simulink model "DaviAraujo_FuelHeatingModel_DashBoardOK"  (R2021a)
settings: Solver=ode5  StartTime=0.0  StopTime=inf  FixedStep=0.01  RelTol=1e-3
values from neighbouring files (symbols this model uses):
  A = 0.0003*4    (= 0.0012)    [FuelHeatingModel_WS.m]
  Densidade_Combustivel = 0.774    [FuelHeatingModel_WS.m]
  EngineTemp = 90    [FuelHeatingModel_WS.m]
  Fluxo_Injetor = 2.141967    [FuelHeatingModel_WS.m]
  h = 12000    [FuelHeatingModel_WS.m]
  Lead_MaxTemp = 80    [FuelHeatingModel_WS.m]
  LeadAcid_TotalEnergy = Voltage_LeadAcid*AmpHour_LeadAcid    (= 600)    [FuelHeatingModel_WS.m]
  Lithium_MaxTemp = 80    [FuelHeatingModel_WS.m]
  Lithium_TotalEnergy = Voltage_Lithium*AmpHour_Lithium    (= 768)    [FuelHeatingModel_WS.m]
  m = (0.4*0.79)    (= 0.316)    [FuelHeatingModel_WS.m]
  Pressure_Ethanol = (P_min:((P_max-P_min)/20):P_max).^4.92    [FuelHeatingModel_WS.m]
  PWM = 0:5:100    [FuelHeatingModel_WS.m]
  RPM_Motor = 1000    [FuelHeatingModel_WS.m]
  Setpoint_ColdStart = 120    [FuelHeatingModel_WS.m]
  Setpoint_PostStart = 90    [FuelHeatingModel_WS.m]
  Temp_Ethanol = 0:6:120    [FuelHeatingModel_WS.m]
  Ts = (Ts_min:((Ts_max-Ts_min)/20):Ts_max).^0.7    [FuelHeatingModel_WS.m]
  VolumeInterno_CommonRail = 7000    [FuelHeatingModel_WS.m]
libraries: simulink x4
(part 1 of 2)
settings Model: NumberOfSteps=10  EnablePacing=on  PacingRate=10  Creator=davi_  LastModifiedBy=davi_
settings SolverCC: AlgebraicLoopSolver=TrustRegion

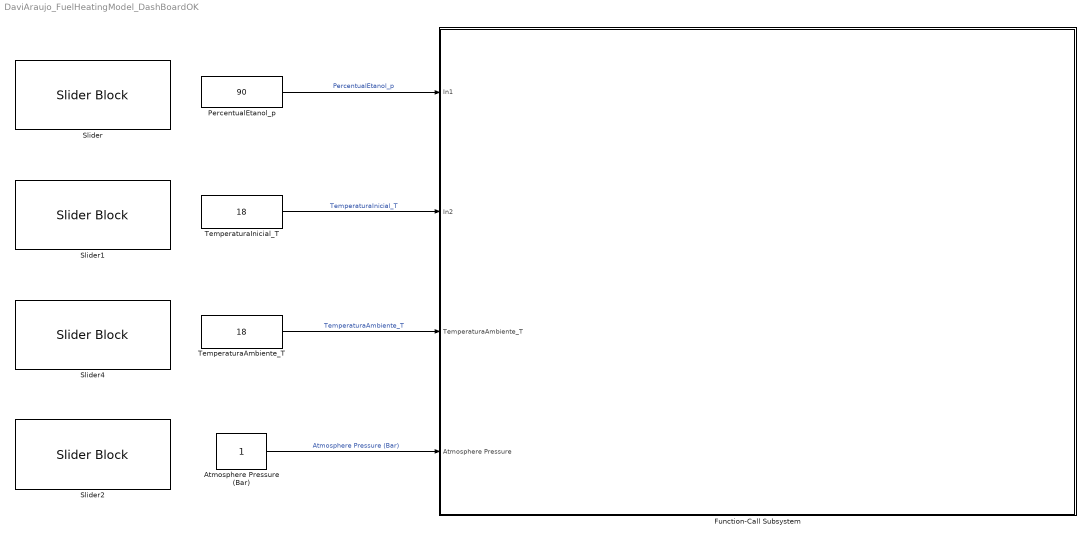
== system DaviAraujo_FuelHeatingModel_DashBoardOK ==
  Atmosphere Pressure (Bar) : Constant
  Function-Call Subsystem : Subsystem  TreatAsAtomicUnit=on
  PercentualEtanol_p : Constant  Value=90
  Slider : SliderBlock
  Slider1 : SliderBlock  ScaleMax=150
  Slider2 : SliderBlock  ScaleMax=2
  Slider4 : SliderBlock  ScaleMin=-20  ScaleMax=40
  TemperaturaAmbiente_T : Constant  Value=18
  TemperaturaInicial_T : Constant  Value=18
  wires:
  Atmosphere Pressure (Bar)/1 -> Function-Call Subsystem/4(Atmosphere Pressure)  "Atmosphere Pressure (Bar)"
  PercentualEtanol_p/1 -> Function-Call Subsystem/1(In1)  "PercentualEtanol_p"
  TemperaturaInicial_T/1 -> Function-Call Subsystem/2(In2)  "TemperaturaInicial_T"
  TemperaturaAmbiente_T/1 -> Function-Call Subsystem/3(TemperaturaAmbiente_T)  "TemperaturaAmbiente_T"

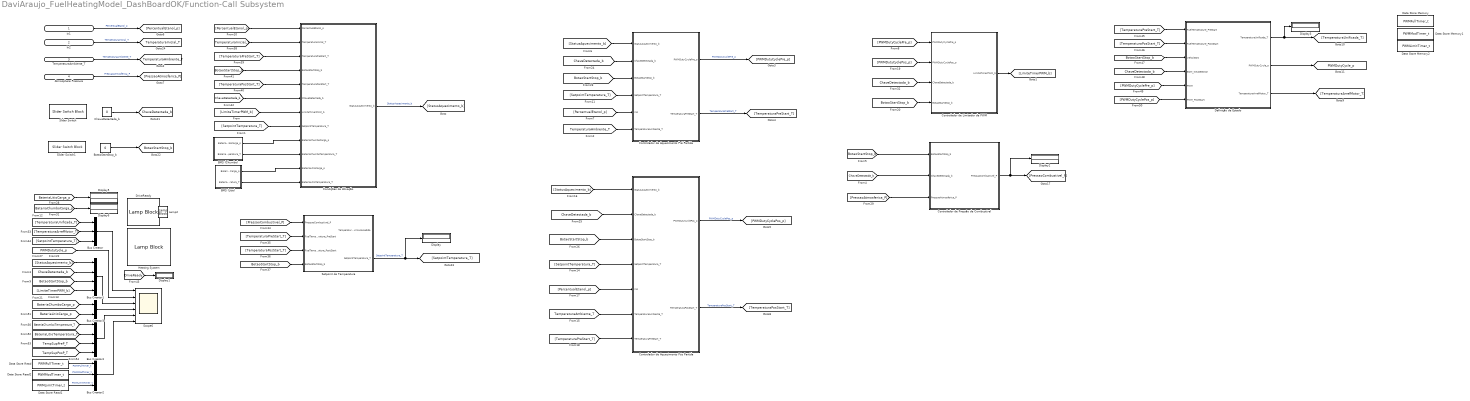
== system DaviAraujo_FuelHeatingModel_DashBoardOK/Function-Call Subsystem ==
  In1 : Inport
  In2 : Inport  Port=2
  TemperaturaAmbiente_T : Inport  Port=3
  Atmosphere Pressure : Inport  Port=4
  BMS (Chumbo) : Subsystem
      mask Display: image('$imagefile'); % Use "Edit Image" on toolstrip to change.
  BMS (Lítio) : Subsystem
      mask Display: image('$imagefile'); % Use "Edit Image" on toolstrip to change.
  BotaoStartStop_b : Constant  Value=0  OutDataTypeStr=boolean
  Bus Creator : BusCreator  Inputs=3
  Bus Creator1 : BusCreator  Inputs=4
  Bus Creator2 : BusCreator  Inputs=3
  Bus Creator3 : BusCreator  Inputs=2
  Bus Creator4 : BusCreator  Inputs=4
  ChaveDetectada_b : Constant  Value=0  OutDataTypeStr=boolean
  Condições de Ativação : Subsystem
  Controlador de Aquecimento Pré Partida : Subsystem
  Controlador de Aquecimento Pós Partida : Subsystem
  Controlador de Limitador de PWM : Subsystem  TreatAsAtomicUnit=on
  Controlador de Pressão de Combustível : Subsystem
  Data Store Memory : DataStoreMemory  DataStoreName=PWMFullTimer_t  ReadBeforeWriteMsg=warning  WriteAfterWriteMsg=warning  WriteAfterReadMsg=warning  ShowAdditionalParam=off
  Data Store Memory1 : DataStoreMemory  DataStoreName=PWMModTimer_t  ReadBeforeWriteMsg=warning  WriteAfterWriteMsg=warning  WriteAfterReadMsg=warning  ShowAdditionalParam=off
  Data Store Memory2 : DataStoreMemory  DataStoreName=PWMLimitTimer_t  ReadBeforeWriteMsg=warning  WriteAfterWriteMsg=warning  WriteAfterReadMsg=warning  ShowAdditionalParam=off
  Data Store Read : DataStoreRead  DataStoreName=PWMFullTimer_t  IndexOptions=Index vector (dialog)  Indices=1  OutputSizes=1
  Data Store Read1 : DataStoreRead  DataStoreName=PWMLimitTimer_t  IndexOptions=Index vector (dialog)  Indices=1  OutputSizes=1
  Data Store Read2 : DataStoreRead  DataStoreName=PWMModTimer_t  IndexOptions=Index vector (dialog)  Indices=1  OutputSizes=1
  Definição de Estado : Subsystem
  Display{,1..3,5..6} (6 alike) : Display
  DriveReady : LampBlock  LabelPosition=Hide  Icon=Check1
  Heating System : LampBlock  LabelPosition=Hide  Icon=Custom  CustomIcon=data:image/svg+xml;base64,PD94bWwgdmVyc2lvbj0iMS4wIiBlbmNvZGluZz0iaXNvLTg4NTktMSI/Pg0KPCEtLSBHZW5lcmF0b3I6IEFkb2JlIElsbHVzdHJhdG9yIDE4LjAuMCwgU1ZHIEV4cG9ydCBQbHVnLUluIC4gU1ZHIFZlcnNpb246IDYuMDAgQnVpbGQgMCkgIC0tPg0KPCFET0NUWVBFIHN2ZyBQVUJMSUMgIi0vL1czQy8vRFREIFNWRyAxLjEvL0VOIiAiaHR0cDovL3d3dy53My5vcmcvR3JhcGhpY3MvU1ZHLzEuMS9EVEQvc3ZnMTEuZHRkIj4NCjxzdmcgdmVyc2lvbj0iMS4xIiBpZD0iQ2FwYV8xIiB4bWxucz0iaHR0cDovL3d3dy53My5vcmcvMjAwMC9zdmciIHhtbG5zOnhsaW5rPSJodHRwOi8vd3d3LnczLm9yZy8xOTk5L3hsaW5rIiB4PSIwcHgiIHk9IjBweCINCgkgdmlld0JveD0iMCAwIDQ2Mi43ODIgNDYyLjc4MiIgc3R5bGU9ImVuYWJsZS1iYWNrZ3JvdW5kOm5ldyAwIDAgNDYyLjc4MiA0NjIuNzgyOyIgeG1sOnNwYWNlPSJwcmVzZXJ2ZSI+DQo8ZyBpZD0iWE1MSURfMjFfIj4NCgk8cGF0aCBpZD0iWE1MSURfOTA0XyIgZD0iTTM1MC4yNzIsMzIzLjAxNGMtNS45NzQsMC0xMS40MTEtMy41NTYtMTMuNzgzLTkuMDkxbC01MC40MjItMTE3LjY1bC00MC41MDUsMTE2LjY2Mg0KCQljLTIuMDgsNS45ODktNy42OTksMTAuMDIzLTE0LjAzOCwxMC4wOGMtMC4wNDQsMC0wLjA4OSwwLTAuMTMzLDBjLTYuMjg2LDAtMTEuOTExLTMuOTIxLTE0LjA4MS05LjgzMWwtNDEuOTc5LTExNC4zNTgNCgkJbC00MC43OTgsMTE0LjIzNGMtMi4wOTUsNS44NjctNy41OTksOS44MjgtMTMuODI3LDkuOTUyYy02LjI0MiwwLjEyNy0xMS44ODYtMy42MTUtMTQuMjEzLTkuMzk0bC0zMS40ODItNzguMTcySDB2LTMwaDg1LjE0MQ0KCQljNi4xMjEsMCwxMS42MjcsMy43MTksMTMuOTE0LDkuMzk2bDIwLjUxMSw1MC45M2w0MS40NDYtMTE2LjA0OGMyLjEyNC01Ljk0Nyw3Ljc0NS05LjkyNywxNC4wNi05Ljk1NWMwLjAyMiwwLDAuMDQ0LDAsMC4wNjYsMA0KCQljNi4yODksMCwxMS45MTIsMy45MjMsMTQuMDgxLDkuODMxbDQxLjc3OSwxMTMuODE0bDM5LjQzMS0xMTMuNTY1YzIuMDMyLTUuODUxLDcuNDUxLTkuODUyLDEzLjY0LTEwLjA3MQ0KCQljNi4yMDMtMC4yMTcsMTEuODc3LDMuMzg5LDE0LjMxNyw5LjA4Mmw0OS42ODMsMTE1LjkyN2wxNS4yNTQtNDguODE1YzEuOTU3LTYuMjYyLDcuNzU2LTEwLjUyNiwxNC4zMTctMTAuNTI2aDg1LjE0MXYzMGgtNzQuMTEzDQoJCWwtMjQuMDc2LDc3LjA0M2MtMS44NzMsNS45OTQtNy4yODEsMTAuMTg2LTEzLjU1MywxMC41MDZDMzUwLjc4NCwzMjMuMDA3LDM1MC41MjcsMzIzLjAxNCwzNTAuMjcyLDMyMy4wMTR6Ii8+DQo8L2c+DQo8Zz4NCjwvZz4NCjxnPg0KPC9nPg0KPGc+DQo8L2c+DQo8Zz4NCjwvZz4NCjxnPg0KPC9nPg0KPGc+DQo8L2c+DQo8Zz4NCjwvZz4NCjxnPg0KPC9nPg0KPGc+DQo8L2c+DQo8Zz4NCjwvZz4NCjxnPg0KPC9nPg0KPGc+DQo8L2c+DQo8Zz4NCjwvZz4NCjxnPg0KPC9nPg0KPGc+DQo8L2c+DQo8L3N2Zz4NCg==
  Lamp2 : LampBlock  LabelPosition=Hide
  Scope6 : Scope  NumInputPorts=6
  Setpoint de Temperatura : Subsystem
  Slider Switch : SliderSwitchBlock
      settings: Values={{'Off', 'On'}, [0 1]}
  Slider Switch1 : SliderSwitchBlock
      settings: Values={{'Off', 'On'}, [0 1]}
  tag scope: BotaoStartStop_b=global, ChaveDetectada_b=global, PWMDutyCycle_p=global, TemperaturaAmbiente_T=global, TemperaturaInicial_T=global
  wires:
  [PWMDutyCyclePre_p] -> Controlador de Limitador de PWM/1(PWMDutyCyclePre_p)
  Controlador de Limitador de PWM/1(LimiteTimerPWM_b) -> [LimiteTimerPWM_b]
  Controlador de Pressão de Combustível/1(PressaoCombustivel_P) -> Display2/1, [PressaoCombustivel_P]
  In1/1 -> [PercentualEtanol_p]  "PercentualEtanol_p"
  [ChaveDetectada_b] -> Controlador de Limitador de PWM/3(ChaveDetectada_b)
  [PressaoCombustivel_P] -> Setpoint de Temperatura/1(PressaoCombustivel_P)
  [TemperaturaPreStart_T] -> Setpoint de Temperatura/2(FuelTemperature_PreStart)
  [TemperaturaPosStart_T] -> Setpoint de Temperatura/3(FuelTemperature_PostStart)
  [BotaoStartStop_b] -> Setpoint de Temperatura/4(BotaoStartStop_b)
  ChaveDetectada_b/1 -> [ChaveDetectada_b]
  BotaoStartStop_b/1 -> [BotaoStartStop_b]
  Setpoint de Temperatura/2(SetpointTemperatura_T) -> Display/1, [SetpointTemperatura_T]  "SetpointTemperatura_T"
  In2/1 -> [TemperaturaInicial_T]  "TemperaturaInicial_T"
  [PercentualEtanol_p] -> Condições de Ativação/1(PercentualEtanol_p)
  [TemperaturaInicial_T] -> Condições de Ativação/2(TemperaturaInicial_T)
  [TemperaturaPreStart_T] -> Condições de Ativação/3(TemperaturaPreStart_T)
  [TemperaturaPosStart_T] -> Condições de Ativação/5(TemperaturaPosStart_T)
  [BotaoStartStop_b] -> Condições de Ativação/4(BotaoStartStop_b)
  [ChaveDetectada_b] -> Condições de Ativação/6(ChaveDetectada_b)
  BMS (Chumbo)/1(BateriaChumboCarga_p) -> Condições de Ativação/9(BateriaChumboCarga_p)
  BMS (Chumbo)/2(BateriaChumboTemperatura_T) -> Condições de Ativação/10(BateriaChumboTemperatura_T)
  BMS (Lítio)/1(BateriaLitioCarga_p) -> Condições de Ativação/11(BateriaLitioCarga_p)
  BMS (Lítio)/2(BateriaLitioTemperatura_T) -> Condições de Ativação/12(BateriaLitioTemperatura_T)
  Condições de Ativação/1(StatusAquecimento_b) -> [StatusAquecimento_b]  "StatusAquecimento_b"
  TemperaturaAmbiente_T/1 -> [TemperaturaAmbiente_T]  "TemperaturaAmbiente_T"
  [StatusAquecimento_b] -> Controlador de Aquecimento Pré Partida/1(StatusAquecimento_b)
  [SetpointTemperatura_T] -> Controlador de Aquecimento Pré Partida/4(SetpointTemperatura_T)
  [PercentualEtanol_p] -> Controlador de Aquecimento Pré Partida/5(In3)
  [BotaoStartStop_b] -> Controlador de Pressão de Combustível/1(BotaoStartStop_b)
  Controlador de Aquecimento Pré Partida/1(PWMDutyCyclePre_p) -> [PWMDutyCyclePre_p]  "PWMDutyCyclePre_p"
  Controlador de Aquecimento Pré Partida/2(TemperaturaPreStart_T) -> [TemperaturaPreStart_T]  "TemperaturaPreStart_T"
  [LimiteTimerPWM_b] -> Condições de Ativação/7(LimiteTimerPWM_b)
  [SetpointTemperatura_T] -> Condições de Ativação/8(SetpointTemperatura_T)
  [TemperaturaAmbiente_T] -> Controlador de Aquecimento Pré Partida/6(TemperaturaAmbiente_T)
  [ChaveDetectada_b] -> Controlador de Pressão de Combustível/2(ChaveDetectada_b)
  [TemperaturaAmbiente_T] -> Controlador de Aquecimento Pós Partida/6(TemperaturaAmbiente_T)
  Controlador de Aquecimento Pós Partida/2(TemperaturaPosStart_T) -> [TemperaturaPosStart_T]  "TemperaturaPosStart_T"
  Controlador de Aquecimento Pós Partida/1(PWMDutyCyclePos_p) -> [PWMDutyCyclePos_p]  "PWMDutyCyclePos_p"
  [PercentualEtanol_p] -> Controlador de Aquecimento Pós Partida/5(In3)
  [StatusAquecimento_b] -> Controlador de Aquecimento Pós Partida/1(StatusAquecimento_b)
  [SetpointTemperatura_T] -> Controlador de Aquecimento Pós Partida/4(SetpointTemperatura_T)
  [TemperaturaPreStart_T] -> Controlador de Aquecimento Pós Partida/7(TemperaturaPreStart_T)
  [PWMDutyCyclePos_p] -> Controlador de Limitador de PWM/2(PWMDutyCyclePos_p)
  [BotaoStartStop_b] -> Controlador de Limitador de PWM/4(BotaoStartStop_b)
  [ChaveDetectada_b] -> Controlador de Aquecimento Pré Partida/2(ChaveDetectada_b)
  [BotaoStartStop_b] -> Controlador de Aquecimento Pré Partida/3(BotaoStartStop_b)
  [ChaveDetectada_b] -> Controlador de Aquecimento Pós Partida/2(ChaveDetectada_b)
  [BotaoStartStop_b] -> Controlador de Aquecimento Pós Partida/3(BotaoStartStop_b)
  [DriveReady] -> Display1/1
  Bus Creator/1 -> Scope6/1
  [BateriaChumboCarga_p] -> Display6/1
  [BateriaLitioCarga_p] -> Display5/1
  [TemperaturaPreStart_T] -> Definição de Estado/1(FuelTemperature_PreStart)
  [TemperaturaPosStart_T] -> Definição de Estado/2(FuelTemperature_PostStart)
  [BotaoStartStop_b] -> Definição de Estado/3(VehicleON)
  [ChaveDetectada_b] -> Definição de Estado/4(BCM_KeyDetector)
  [PWMDutyCyclePre_p] -> Definição de Estado/5(PWM)
  [PWMDutyCyclePos_p] -> Definição de Estado/6(PWM_PostStart)
  Definição de Estado/1(TemperaturaUnificada_T) -> Display3/1, [TemperaturaUnificada_T]
  Definição de Estado/2(PWMDutyCycle_p) -> [PWMDutyCycle_p]
  Atmosphere Pressure/1 -> [PressaoAtmosferica_P]  "PressaoAtmosferica_P"
  [PressaoAtmosferica_P] -> Controlador de Pressão de Combustível/3(PressaoAtmosferica_P)
  Definição de Estado/3(TemperaturaArrefMotor_T) -> [TemperaturaArrefMotor_T]
  [TemperaturaUnificada_T] -> Bus Creator/1
  [TemperaturaArrefMotor_T] -> Bus Creator/2
  [SetpointTemperatura_T] -> Bus Creator/3
  [StatusAquecimento_b] -> Bus Creator1/1
  [ChaveDetectada_b] -> Bus Creator1/2
  [BotaoStartStop_b] -> Bus Creator1/3
  [LimiteTimerPWM_b] -> Bus Creator1/4
  [BateriaChumboCarga_p] -> Bus Creator3/1
  Bus Creator3/1 -> Scope6/4
  Bus Creator2/1 -> Scope6/6
  Data Store Read/1 -> Bus Creator2/1  "PWMFullTimer_t"
  Data Store Read2/1 -> Bus Creator2/2  "PWMModTimer_t"
  Data Store Read1/1 -> Bus Creator2/3  "PWMLimitTimer_t"
  [BateriaLitioCarga_p] -> Bus Creator3/2
  [BateriaChumboTemperatura_T] -> Bus Creator4/1
  [BateriaLitioTemperatura_T] -> Bus Creator4/2
  Bus Creator4/1 -> Scope6/5
  [PWMDutyCycle_p] -> Scope6/2
  Bus Creator1/1 -> Scope6/3
  [TempSupPreP_T] -> Bus Creator4/3
  [TempSupPosP_T] -> Bus Creator4/4

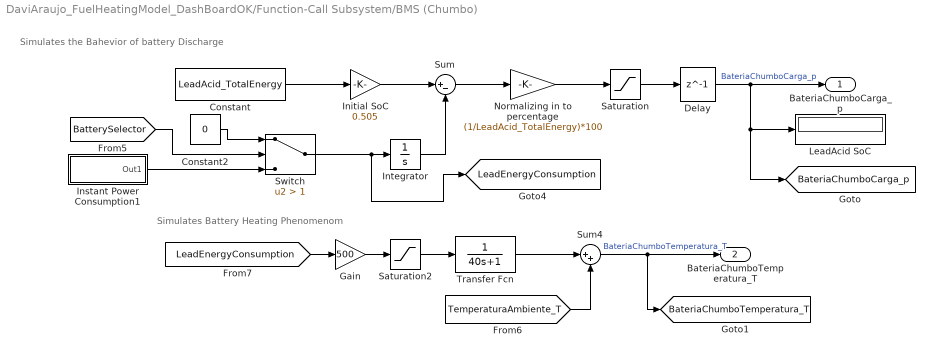
== system DaviAraujo_FuelHeatingModel_DashBoardOK/Function-Call Subsystem/BMS (Chumbo) ==
  note: Simulates Battery Heating Phenomenom
  note: Simulates the Bahevior of battery Discharge
  Constant : Constant  Value=LeadAcid_TotalEnergy
  Constant2 : Constant  Value=0
  Delay : Delay  DelayLength=1  InitialCondition=100  SampleTime=0.01
  Gain : Gain  Gain=500
  Initial SoC : Gain  Gain=0.505
  Instant Power Consumption1 : Subsystem
  Integrator : Integrator
  LeadAcid SoC : Display
  Normalizing in to percentage : Gain  Gain=(1/LeadAcid_TotalEnergy)*100
  Saturation : Saturate  UpperLimit=100  LowerLimit=0
  Saturation2 : Saturate  UpperLimit=120  LowerLimit=-inf
  Sum : Sum  Inputs=|+-
  Sum4 : Sum  Inputs=|++
  Switch : Switch  Criteria=u2 > Threshold  Threshold=1
  Transfer Fcn : TransferFcn  Denominator=[40 1]
  BateriaChumboCarga_p : Outport  VectorParamsAs1DForOutWhenUnconnected=off
  BateriaChumboTemperatura_T : Outport  Port=2  VectorParamsAs1DForOutWhenUnconnected=off
  tag scope: BateriaChumboCarga_p=global, BateriaChumboTemperatura_T=global, LeadEnergyConsumption=global
  wires:
  [LeadEnergyConsumption] -> Gain/1
  Saturation2/1 -> Transfer Fcn/1
  [TemperaturaAmbiente_T] -> Sum4/2
  Sum4/1 -> BateriaChumboTemperatura_T/1, [BateriaChumboTemperatura_T]  "BateriaChumboTemperatura_T"
  Gain/1 -> Saturation2/1
  Transfer Fcn/1 -> Sum4/1
  Switch/1 -> [LeadEnergyConsumption], Integrator/1
  Instant Power Consumption1/1(Out1) -> Switch/3
  Constant2/1 -> Switch/1
  [BatterySelector] -> Switch/2
  Constant/1 -> Initial SoC/1
  Delay/1 -> [BateriaChumboCarga_p], LeadAcid SoC/1, BateriaChumboCarga_p/1  "BateriaChumboCarga_p"
  Sum/1 -> Normalizing in to percentage/1
  Normalizing in to percentage/1 -> Saturation/1
  Initial SoC/1 -> Sum/1
  Integrator/1 -> Sum/2
  Saturation/1 -> Delay/1

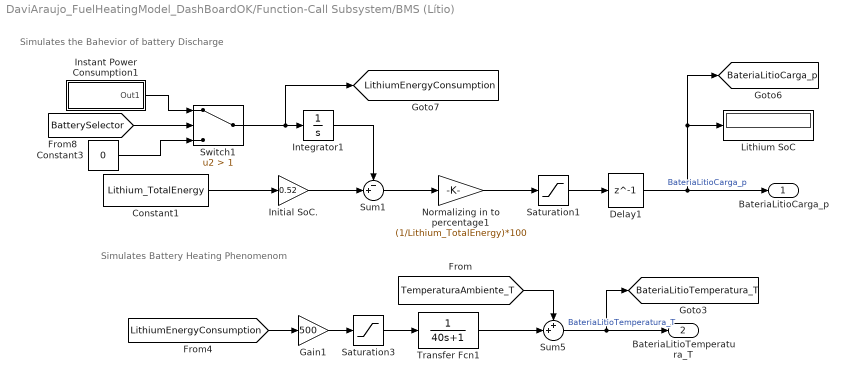
== system DaviAraujo_FuelHeatingModel_DashBoardOK/Function-Call Subsystem/BMS (Lítio) ==
  note: Simulates Battery Heating Phenomenom
  note: Simulates the Bahevior of battery Discharge
  Constant1 : Constant  Value=Lithium_TotalEnergy
  Constant3 : Constant  Value=0
  Delay1 : Delay  DelayLength=1  InitialCondition=100  SampleTime=0.01
  Gain1 : Gain  Gain=500
  Initial SoC. : Gain  Gain=0.52
  Instant Power Consumption1 : Subsystem
  Integrator1 : Integrator
  Lithium SoC : Display
  Normalizing in to percentage1 : Gain  Gain=(1/Lithium_TotalEnergy)*100
  Saturation1 : Saturate  UpperLimit=100  LowerLimit=0
  Saturation3 : Saturate  UpperLimit=120  LowerLimit=-inf
  Sum1 : Sum  Inputs=-+|
  Sum5 : Sum  Inputs=++|
  Switch1 : Switch  Criteria=u2 > Threshold  Threshold=1
  Transfer Fcn1 : TransferFcn  Denominator=[40 1]
  BateriaLitioCarga_p : Outport  VectorParamsAs1DForOutWhenUnconnected=off
  BateriaLitioTemperatura_T : Outport  Port=2  VectorParamsAs1DForOutWhenUnconnected=off
  tag scope: BateriaLitioCarga_p=global, BateriaLitioTemperatura_T=global, LithiumEnergyConsumption=global
  wires:
  [LithiumEnergyConsumption] -> Gain1/1
  Gain1/1 -> Saturation3/1
  [TemperaturaAmbiente_T] -> Sum5/1
  Sum5/1 -> BateriaLitioTemperatura_T/1, [BateriaLitioTemperatura_T]  "BateriaLitioTemperatura_T"
  Transfer Fcn1/1 -> Sum5/2
  Saturation3/1 -> Transfer Fcn1/1
  [BatterySelector] -> Switch1/2
  Normalizing in to percentage1/1 -> Saturation1/1
  Saturation1/1 -> Delay1/1
  Instant Power Consumption1/1(Out1) -> Switch1/1
  Delay1/1 -> BateriaLitioCarga_p/1, [BateriaLitioCarga_p], Lithium SoC/1  "BateriaLitioCarga_p"
  Initial SoC./1 -> Sum1/2
  Constant1/1 -> Initial SoC./1
  Switch1/1 -> [LithiumEnergyConsumption], Integrator1/1
  Integrator1/1 -> Sum1/1
  Constant3/1 -> Switch1/3
  Sum1/1 -> Normalizing in to percentage1/1

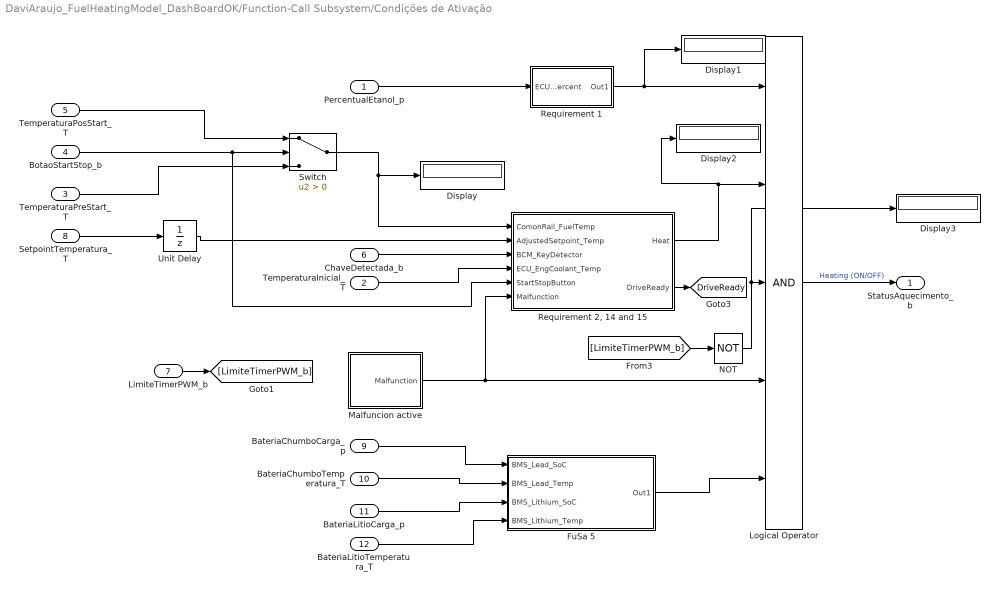
== system DaviAraujo_FuelHeatingModel_DashBoardOK/Function-Call Subsystem/Condições de Ativação ==
  PercentualEtanol_p : Inport
  TemperaturaInicial_T : Inport  Port=2
  TemperaturaPreStart_T : Inport  Port=3
  BotaoStartStop_b : Inport  Port=4
  TemperaturaPosStart_T : Inport  Port=5
  ChaveDetectada_b : Inport  Port=6
  LimiteTimerPWM_b : Inport  Port=7
  SetpointTemperatura_T : Inport  Port=8
  BateriaChumboCarga_p : Inport  Port=9
  BateriaChumboTemperatura_T : Inport  Port=10
  BateriaLitioCarga_p : Inport  Port=11
  BateriaLitioTemperatura_T : Inport  Port=12
  Display{,1..3} (4 alike) : Display
  FuSa 5 : Subsystem
  Logical Operator : Logic  Inputs=5  AllPortsSameDT=off  OutDataTypeStr=boolean
  Malfuncion active : Subsystem
  NOT : Logic  Operator=NOT  IconShape=distinctive  AllPortsSameDT=off  OutDataTypeStr=boolean
  "Requirement 1 " : Subsystem
  "Requirement 2, 14 and 15" : Stateflow chart  TreatAsAtomicUnit=on
  Switch : Switch  Criteria=u2 > Threshold
  Unit Delay : UnitDelay  SampleTime=-1  HasFrameUpgradeWarning=on
  StatusAquecimento_b : Outport
  tag scope: DriveReady=global
  wires:
  "Requirement 1 "/1(Out1) -> Display1/1, Logical Operator/1
  Logical Operator/1 -> StatusAquecimento_b/1  "Heating (ON/OFF)"
  SetpointTemperatura_T/1 -> Unit Delay/1
  "Requirement 2, 14 and 15"/1(Heat) -> Display2/1, Logical Operator/2
  [LimiteTimerPWM_b] -> NOT/1
  "Requirement 2, 14 and 15"/2(DriveReady) -> [DriveReady]
  FuSa 5/1(Out1) -> Logical Operator/5
  PercentualEtanol_p/1 -> "Requirement 1 "/1(ECU_EthanolPercent)
  BateriaLitioTemperatura_T/1 -> FuSa 5/4(BMS_Lithium_Temp)
  BateriaChumboCarga_p/1 -> FuSa 5/1(BMS_Lead_SoC)
  BateriaChumboTemperatura_T/1 -> FuSa 5/2(BMS_Lead_Temp)
  BateriaLitioCarga_p/1 -> FuSa 5/3(BMS_Lithium_SoC)
  ChaveDetectada_b/1 -> "Requirement 2, 14 and 15"/3(BCM_KeyDetector)
  TemperaturaInicial_T/1 -> "Requirement 2, 14 and 15"/4(ECU_EngCoolant_Temp)
  Malfuncion active/1(Malfunction) -> Logical Operator/4, "Requirement 2, 14 and 15"/6(Malfunction)
  LimiteTimerPWM_b/1 -> [LimiteTimerPWM_b]
  Unit Delay/1 -> "Requirement 2, 14 and 15"/2(AdjustedSetpoint_Temp)
  BotaoStartStop_b/1 -> "Requirement 2, 14 and 15"/5(StartStopButton), Switch/2
  TemperaturaPosStart_T/1 -> Switch/1
  Switch/1 -> Display/1, "Requirement 2, 14 and 15"/1(ComonRail_FuelTemp)
  TemperaturaPreStart_T/1 -> Switch/3
  NOT/1 -> Logical Operator/3, Display3/1

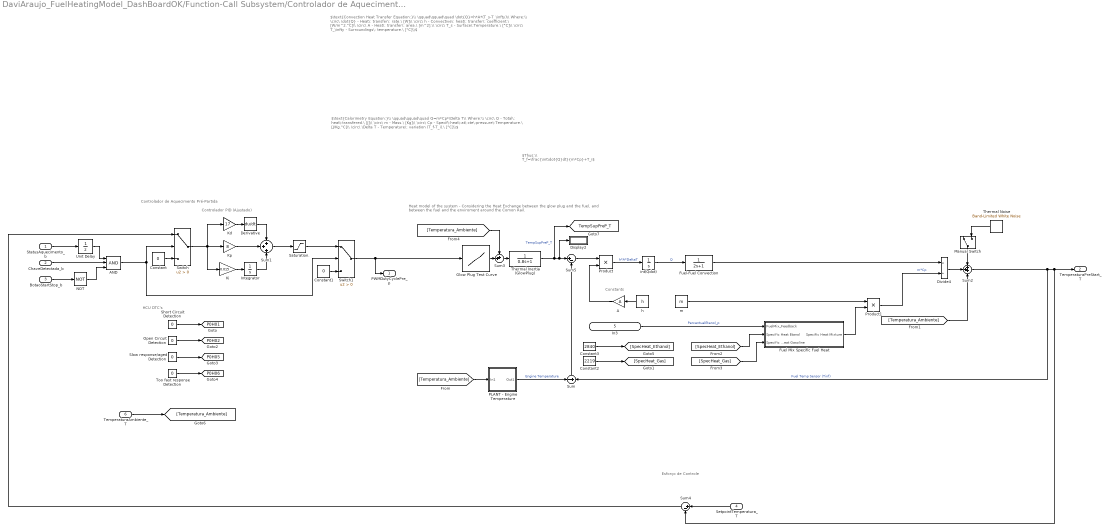
== system DaviAraujo_FuelHeatingModel_DashBoardOK/Function-Call Subsystem/Controlador de Aquecimento Pré Partida ==
  note: Esforço de Controle
  note: Controlador de Aquecimento Pré-Partida
  note: Controlador PID (Ajustado)
  note: HCU DTC's
  note: Constants
  note: $\text{Calorimetry Equation:}\\ \qquad\qquad\quad Q=m*Cp*\Delta T\\ Where:\\ \circ\ Q - Total\: heat\:transfered.\ [J]\\ \circ\ m - Mass.\ [Kg]\\ \circ\ Cp - Specif\:heat\:at\:cte\:pressure\:Temperature.\ [J/Kg.°C]\\ \circ\ \Delta T - Temperature\: variation (T_f-T_i).\ [°C]\\$
  note: $\text{Convection Heat Transfer Equation:}\\ \qquad\qquad\quad \dot{Q}=h*A*(T_s-T_\infty)\\ Where:\\ \circ\ \dot{Q} - Heat\: transfer\: rate.\ [W]\\ \circ\ h - Convective\: heat\: transfer\: coefficient.\ [W/m^2.°C]\\ \circ\ A - Heat\: transfer\: area.\ [m^2].\\ \circ\ T_s - Surface\:Temperature.\ [°C]\\ \circ\ T_\infty - Surroundings\: temperature.\ [°C]\\$
  note: Heat model of the system - Considering the Heat Exchange between the glow plug and the fuel, and between the fuel and the enviroment around the Comon Rail.
  note: $Thus:\\ T_f=\frac{\int\dot{Q}dt}{m*Cp}+T_i$
  StatusAquecimento_b : Inport
  ChaveDetectada_b : Inport  Port=2
  BotaoStartStop_b : Inport  Port=3
  SetpointTemperatura_T : Inport  Port=4
  In3 : Inport  Port=5
  TemperaturaAmbiente_T : Inport  Port=6
  A : Gain  Gain=A
  AND : Logic  Inputs=3  IconShape=distinctive  AllPortsSameDT=off  OutDataTypeStr=boolean
  Constant : Constant  Value=0
  Constant1 : Constant  Value=0
  Constant2 : Constant  Value=2219
  Constant3 : Constant  Value=2840
  Derivative : Derivative
  Display2 : Display
  Divide4 : Product  Inputs=*/
  Fuel Mix Specific Fuel Heat : Subsystem
  Fuel-Fuel Convection : TransferFcn  Denominator=[2 1]
  Glow Plug Test Curve : Lookup_n-D  NumberOfTableDimensions=1  BreakpointsForDimension1=PWM  BreakpointsForDimension2=[1:3]  Table=Ts  InternalRulePriority=Speed  RndMeth=Simplest  InputSameDT=on
  Integrator : Integrator
  Kd : Gain  Gain=17
  Ki : Gain  Gain=0.015
  Kp : Gain  Gain=8
  Manual Switch : ManualSwitch
  NOT : Logic  Operator=NOT  IconShape=distinctive  AllPortsSameDT=off  OutDataTypeStr=boolean
  Open Circuit Detection : Constant  Value=0
  PLANT - Engine Temperature : Subsystem
  Product : Product
  Product1 : Product
  Saturation. : Saturate  UpperLimit=100  LowerLimit=0
  Short Circuit Detection : Constant  Value=0
  Slow response/aged Detection : Constant  Value=0
  Sum : Sum  Inputs=-+
  Sum1 : Sum  Inputs=+++
  Sum2 : Sum  Inputs=+++
  Sum3 : Sum  Inputs=++|
  Sum4 : Sum  Inputs=|+-
  Sum5 : Sum  Inputs=|+-
  Switch : Switch  Criteria=u2 > Threshold
  Switch1 : Switch  Criteria=u2 > Threshold
  Thermal Inertia (GlowPlug) : TransferFcn  Denominator=[0.8 1]
  Thermal Noise : simulink/Sources/Band-Limited White Noise  Cov=[0.001]  Ts=0.05  seed=[23341]
  Too fast response Detection : Constant  Value=0
  Unit Delay : UnitDelay  SampleTime=-1  HasFrameUpgradeWarning=on
  h : Constant  Value=h
  int(Qdot) : Integrator
  m : Constant  Value=m
  PWMDutyCyclePre_p : Outport
  TemperaturaPreStart_T : Outport  Port=2  VectorParamsAs1DForOutWhenUnconnected=off
  tag scope: P0H01=global, P0H02=global, P0H05=global, P0H06=global, TempSupPreP_T=global
  wires:
  Constant/1 -> Switch/3
  StatusAquecimento_b/1 -> Unit Delay/1
  Saturation./1 -> Switch1/1
  Derivative/1 -> Sum1/1
  Ki/1 -> Integrator/1
  Kd/1 -> Derivative/1
  Kp/1 -> Sum1/2
  Constant1/1 -> Switch1/3
  Integrator/1 -> Sum1/3
  Short Circuit Detection/1 -> [P0H01]
  Too fast response Detection/1 -> [P0H06]
  Slow response/aged Detection/1 -> [P0H05]
  Open Circuit Detection/1 -> [P0H02]
  [Temperatura_Ambiente] -> Sum3/1
  Glow Plug Test Curve/1 -> Sum3/2
  Manual Switch/1 -> Sum2/1
  int(Qdot)/1 -> Fuel-Fuel Convection/1  "Q"
  Divide4/1 -> Sum2/2
  Sum5/1 -> Product/1
  Sum/1 -> Sum5/2
  A/1 -> Product/2
  Sum3/1 -> Thermal Inertia (GlowPlug)/1
  Product/1 -> int(Qdot)/1  "h*A*DeltaT"
  PLANT - Engine Temperature/1(Out1) -> Sum/1  "Engine Temperature"
  h/1 -> A/1
  Thermal Noise/1 -> Manual Switch/2
  Thermal Inertia (GlowPlug)/1 -> [TempSupPreP_T], Display2/1, Sum5/1  "TempSupPreP_T"
  Fuel-Fuel Convection/1 -> Divide4/1
  Sum2/1 -> TemperaturaPreStart_T/1, Sum4/2, Sum/2  "Fuel Temp Sensor (Tinf)"
  m/1 -> Product1/1
  Switch1/1 -> PWMDutyCyclePre_p/1, Glow Plug Test Curve/1
  SetpointTemperatura_T/1 -> Sum4/1
  Sum4/1 -> Switch/1
  In3/1 -> Fuel Mix Specific Fuel Heat/1(FuelMix_Feedback)  "PercentualEtanol_p"
  Constant2/1 -> [SpecHeat_Gas]
  [SpecHeat_Gas] -> Fuel Mix Specific Fuel Heat/3(Specific Heat Gasoline)
  Constant3/1 -> [SpecHeat_Ethanol]
  [SpecHeat_Ethanol] -> Fuel Mix Specific Fuel Heat/2(Specific Heat Etanol)
  Fuel Mix Specific Fuel Heat/1(Specific Heat Mixture) -> Product1/2
  Product1/1 -> Divide4/2  "m*Cp"
  TemperaturaAmbiente_T/1 -> [Temperatura_Ambiente]
  AND/1 -> Switch1/2, Switch/2
  Unit Delay/1 -> AND/1
  ChaveDetectada_b/1 -> AND/2
  BotaoStartStop_b/1 -> NOT/1
  Switch/1 -> Ki/1, Kp/1, Kd/1
  Sum1/1 -> Saturation./1
  [Temperatura_Ambiente] -> PLANT - Engine Temperature/1(In1)
  NOT/1 -> AND/3
  [Temperatura_Ambiente] -> Sum2/3

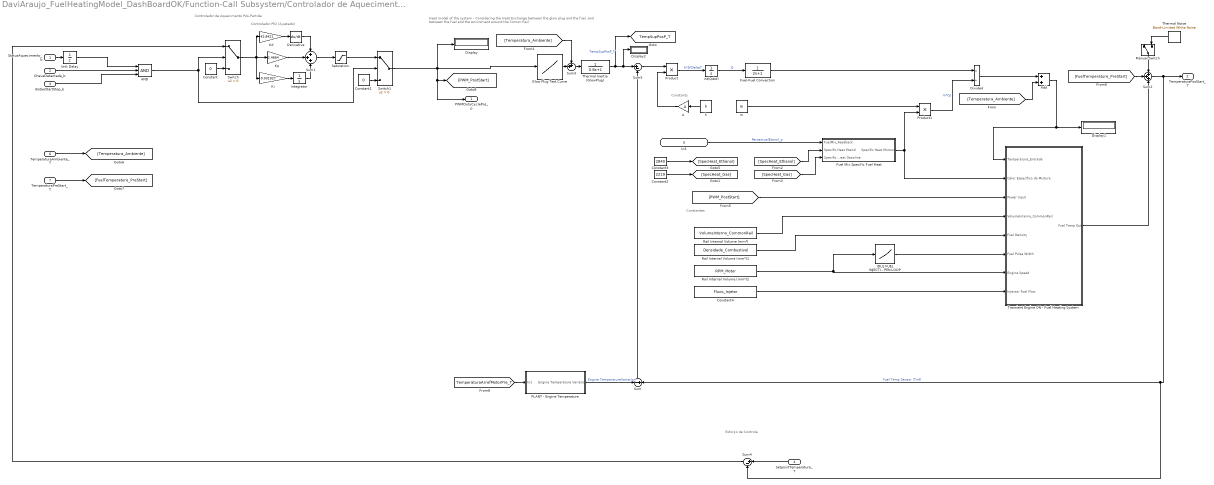
== system DaviAraujo_FuelHeatingModel_DashBoardOK/Function-Call Subsystem/Controlador de Aquecimento Pós Partida ==
  note: Constantes
  note: Esforço de Controle
  note: Controlador de Aquecimento Pós-Partida
  note: Controlador PID (Ajustado)
  note: Heat model of the system - Considering the Heat Exchange between the glow plug and the fuel, and between the fuel and the enviroment around the Comon Rail.
  note: Constants
  StatusAquecimento_b : Inport
  ChaveDetectada_b : Inport  Port=2
  BotaoStartStop_b : Inport  Port=3
  SetpointTemperatura_T : Inport  Port=4
  In3 : Inport  Port=5
  TemperaturaAmbiente_T : Inport  Port=6
  TemperaturaPreStart_T : Inport  Port=7
  A : Gain  Gain=A
  AND : Logic  Inputs=3  IconShape=distinctive  AllPortsSameDT=off  OutDataTypeStr=boolean
  Add : Sum
  Constant : Constant  Value=0
  Constant1 : Constant  Value=0
  Constant2 : Constant  Value=2219
  Constant3 : Constant  Value=2840
  Constant4 : Constant  Value=Fluxo_Injetor
  Derivative : Derivative
  Display : Display
  Display1 : Display
  Display2 : Display
  Divide4 : Product  Inputs=*/
  Fuel Mix Specific Fuel Heat : Subsystem
  Fuel-Fuel Convection : TransferFcn  Denominator=[2 1]
  Glow Plug Test Curve : Lookup_n-D  NumberOfTableDimensions=1  BreakpointsForDimension1=PWM  BreakpointsForDimension2=[1:3]  Table=Ts  InternalRulePriority=Speed  RndMeth=Simplest  InputSameDT=on
  IDLE FUEL INJECTION TABLE OPEN LOOP : Lookup_n-D  NumberOfTableDimensions=1  BreakpointsForDimension1=[900 1500 1800 2000 2200 2500 2700 3200]  Table=[5.003 2.66 2.407 2.76 2.606 2.826 3.607 3.601]  InternalRulePriority=Speed  RndMeth=Simplest  InputSameDT=on
  Integrator : Integrator
  Kd : Gain  Gain=42.8421
  Ki : Gain  Gain=0.031927
  Kp : Gain  Gain=2.4664
  Manual Switch : ManualSwitch
  PLANT - Engine Temperature : Subsystem
  Product : Product
  Product1 : Product
  Rail Internal Volume (mm³) : Constant  Value=VolumeInterno_CommonRail
  Rail Internal Volume (mm³)1 : Constant  Value=Densidade_Combustivel
  Rail Internal Volume (mm³)2 : Constant  Value=RPM_Motor
  Saturation. : Saturate  UpperLimit=100  LowerLimit=0
  Sum : Sum  Inputs=-+
  Sum1 : Sum  Inputs=+++
  Sum2 : Sum  Inputs=+++
  Sum3 : Sum  Inputs=++|
  Sum4 : Sum  Inputs=|+-
  Sum5 : Sum  Inputs=|+-
  Switch : Switch  Criteria=u2 > Threshold
  Switch1 : Switch  Criteria=u2 > Threshold
  Thermal Inertia (GlowPlug) : TransferFcn  Denominator=[0.8 1]
  Thermal Noise : simulink/Sources/Band-Limited White Noise  Cov=[0.001]  Ts=0.05  seed=[23341]
  Transient Engine ON - Fuel Heating System : Subsystem
  Unit Delay : UnitDelay  SampleTime=-1  HasFrameUpgradeWarning=on
  h : Constant  Value=h
  int(Qdot) : Integrator
  m : Constant  Value=m
  PWMDutyCyclePos_p : Outport
  TemperaturaPosStart_T : Outport  Port=2  VectorParamsAs1DForOutWhenUnconnected=off
  tag scope: TempSupPosP_T=global
  wires:
  Constant/1 -> Switch/3
  StatusAquecimento_b/1 -> Unit Delay/1
  Derivative/1 -> Sum1/1
  Ki/1 -> Integrator/1
  Kd/1 -> Derivative/1
  Kp/1 -> Sum1/2
  Constant1/1 -> Switch1/3
  Integrator/1 -> Sum1/3
  [Temperatura_Ambiente] -> Sum3/1
  Glow Plug Test Curve/1 -> Sum3/2
  Manual Switch/1 -> Sum2/1
  Sum/1 -> Sum5/2
  Sum3/1 -> Thermal Inertia (GlowPlug)/1
  PLANT - Engine Temperature/1(Engine Temperature Variation) -> Sum/1  "Engine TemperatureVariation"
  Thermal Noise/1 -> Manual Switch/2
  Thermal Inertia (GlowPlug)/1 -> [TempSupPosP_T], Sum5/1, Display2/1  "TempSupPosP_T"
  Sum2/1 -> TemperaturaPosStart_T/1, Sum/2, Sum4/2  "Fuel Temp Sensor (Tinf)"
  Switch1/1 -> Display/1, Glow Plug Test Curve/1, PWMDutyCyclePos_p/1, [PWM_PostStart]
  SetpointTemperatura_T/1 -> Sum4/1
  Sum4/1 -> Switch/1
  In3/1 -> Fuel Mix Specific Fuel Heat/1(FuelMix_Feedback)  "PercentualEtanol_p"
  Constant2/1 -> [SpecHeat_Gas]
  [SpecHeat_Gas] -> Fuel Mix Specific Fuel Heat/3(Specific Heat Gasoline)
  Constant3/1 -> [SpecHeat_Ethanol]
  [SpecHeat_Ethanol] -> Fuel Mix Specific Fuel Heat/2(Specific Heat Etanol)
  TemperaturaAmbiente_T/1 -> [Temperatura_Ambiente]
  Rail Internal Volume (mm³)2/1 -> Transient Engine ON - Fuel Heating System/7(Engine Speed), IDLE FUEL INJECTION TABLE OPEN LOOP/1
  Constant4/1 -> Transient Engine ON - Fuel Heating System/8(Injector Fuel Flow)
  Rail Internal Volume (mm³)1/1 -> Transient Engine ON - Fuel Heating System/5(Fuel Density)
  Rail Internal Volume (mm³)/1 -> Transient Engine ON - Fuel Heating System/4(VolumeInterno_CommonRail)
  TemperaturaPreStart_T/1 -> [FuelTemperature_PreStart]
  [PWM_PostStart] -> Transient Engine ON - Fuel Heating System/3(Power Input)
  IDLE FUEL INJECTION TABLE OPEN LOOP/1 -> Transient Engine ON - Fuel Heating System/6(Fuel Pulse Width)
  Transient Engine ON - Fuel Heating System/1(Fuel Temp Out) -> Sum2/3
  Unit Delay/1 -> AND/1
  ChaveDetectada_b/1 -> AND/2
  BotaoStartStop_b/1 -> AND/3
  AND/1 -> Switch1/2, Switch/2
  Fuel Mix Specific Fuel Heat/1(Specific Heat Mixture) -> Transient Engine ON - Fuel Heating System/2(Calor Específico da Mistura), Product1/2
  Product1/1 -> Divide4/2  "m*Cp"
  h/1 -> A/1
  A/1 -> Product/2
  int(Qdot)/1 -> Fuel-Fuel Convection/1  "Q"
  m/1 -> Product1/1
  Product/1 -> int(Qdot)/1  "h*A*DeltaT"
  Fuel-Fuel Convection/1 -> Divide4/1
  Sum5/1 -> Product/1
  Divide4/1 -> Add/1
  [Temperatura_Ambiente] -> Add/2
  Add/1 -> Display1/1, Transient Engine ON - Fuel Heating System/1(Temperatura_Entrada)
  Switch/1 -> Ki/1, Kp/1, Kd/1
  Sum1/1 -> Saturation./1
  Saturation./1 -> Switch1/1
  [FuelTemperature_PreStart] -> Sum2/2
  [TemperaturaArrefMotorPre_T] -> PLANT - Engine Temperature/1(In1)

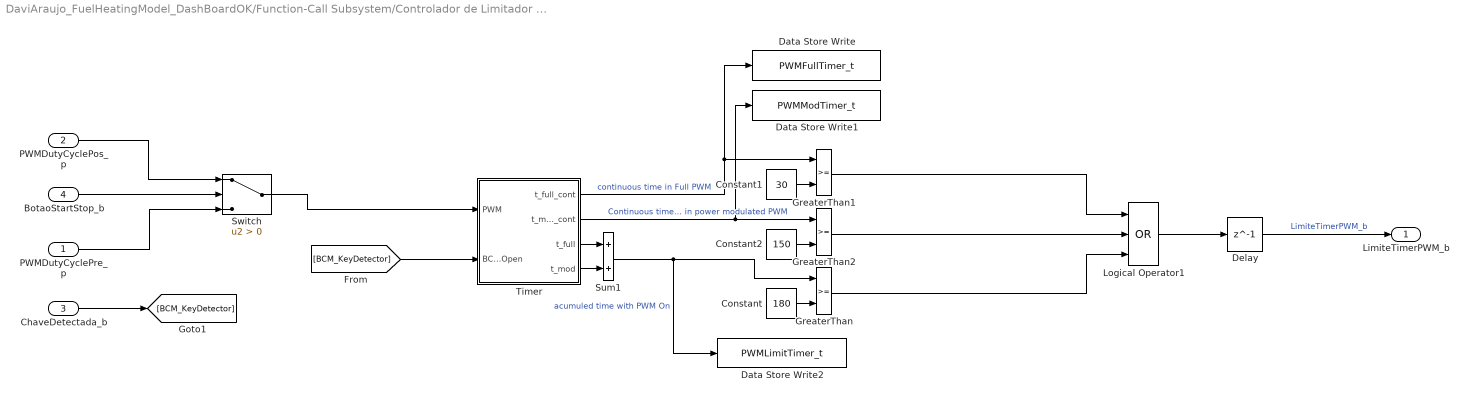
== system DaviAraujo_FuelHeatingModel_DashBoardOK/Function-Call Subsystem/Controlador de Limitador de PWM ==
  PWMDutyCyclePre_p : Inport
  PWMDutyCyclePos_p : Inport  Port=2
  ChaveDetectada_b : Inport  Port=3
  BotaoStartStop_b : Inport  Port=4
  Constant : Constant  Value=180
  Constant1 : Constant  Value=30
  Constant2 : Constant  Value=150
  Data Store Write : DataStoreWrite  DataStoreName=PWMFullTimer_t  IndexOptions=Index vector (dialog)  Indices=1  OutputSizes=1
  Data Store Write1 : DataStoreWrite  DataStoreName=PWMModTimer_t  IndexOptions=Index vector (dialog)  Indices=1  OutputSizes=1
  Data Store Write2 : DataStoreWrite  DataStoreName=PWMLimitTimer_t  IndexOptions=Index vector (dialog)  Indices=1  OutputSizes=1
  Delay : Delay  DelayLength=1  InitialCondition=0  SampleTime=0.01
  GreaterThan : RelationalOperator  OutDataTypeStr=boolean  RndMeth=Simplest
  GreaterThan1 : RelationalOperator  OutDataTypeStr=boolean  RndMeth=Simplest
  GreaterThan2 : RelationalOperator  OutDataTypeStr=boolean  RndMeth=Simplest
  Logical Operator1 : Logic  Operator=OR  Inputs=3  AllPortsSameDT=off  OutDataTypeStr=boolean
  Sum1 : Sum
  Switch : Switch  Criteria=u2 > Threshold
  Timer : Stateflow chart  TreatAsAtomicUnit=on
  LimiteTimerPWM_b : Outport
  wires:
  [BCM_KeyDetector] -> Timer/2(BCM_DoorOpen)
  Timer/2(t_mod_cont) -> Data Store Write1/1, GreaterThan2/1  "Continuous time in power modulated PWM"
  Timer/1(t_full_cont) -> Data Store Write/1, GreaterThan1/1  "continuous time in Full PWM"
  Constant/1 -> GreaterThan/2
  Timer/4(t_mod) -> Sum1/2
  Sum1/1 -> Data Store Write2/1, GreaterThan/1  "acumuled time with PWM On"
  Constant1/1 -> GreaterThan1/2
  Timer/3(t_full) -> Sum1/1
  Constant2/1 -> GreaterThan2/2
  ChaveDetectada_b/1 -> [BCM_KeyDetector]
  GreaterThan2/1 -> Logical Operator1/2
  Delay/1 -> LimiteTimerPWM_b/1  "LimiteTimerPWM_b"
  Logical Operator1/1 -> Delay/1
  GreaterThan/1 -> Logical Operator1/3
  GreaterThan1/1 -> Logical Operator1/1
  BotaoStartStop_b/1 -> Switch/2
  PWMDutyCyclePos_p/1 -> Switch/1
  PWMDutyCyclePre_p/1 -> Switch/3
  Switch/1 -> Timer/1(PWM)

== system DaviAraujo_FuelHeatingModel_DashBoardOK/Function-Call Subsystem/Controlador de Pressão de Combustível ==
  BotaoStartStop_b : Inport
  ChaveDetectada_b : Inport  Port=2
  PressaoAtmosferica_P : Inport  Port=3
  1-D Lookup Table2 : Lookup_n-D  NumberOfTableDimensions=1  BreakpointsForDimension1=[0 0.000001 0.000002 3 3.00001 10 10.0001 13 13.0001 20]  Table=[0 0 1 1 1 1 1 1 1 1]  InternalRulePriority=Speed  RndMeth=Simplest  InputSameDT=on
  1-D Lookup Table3 : Lookup_n-D  NumberOfTableDimensions=1  BreakpointsForDimension1=[0 0.000001 0.000002 3 3.00001 10 10.0001 13 13.0001 20]  Table=[0 0 1 1 0 0 0 0 0 0]  InternalRulePriority=Speed  RndMeth=Simplest  InputSameDT=on
  Clock : Clock
  Clock1 : Clock
  EngineOFF_PressureController1 : Subsystem
  EngineON_PressureController1 : Subsystem
  Switch : Switch  Criteria=u2 ~= 0
  Switch1 : Switch  Criteria=u2 ~= 0
  PressaoCombustivel_P : Outport
  wires:
  PressaoAtmosferica_P/1 -> Switch1/3, EngineON_PressureController1/2(Atmosphere Pressure), EngineOFF_PressureController1/2(Atmosphere Pressure)
  EngineOFF_PressureController1/1(Out1) -> Switch/1
  EngineON_PressureController1/1(Out1) -> Switch/3
  1-D Lookup Table2/1 -> EngineON_PressureController1/1(PUMP SIGNAL 1 - ON)
  Clock/1 -> 1-D Lookup Table2/1
  Clock1/1 -> 1-D Lookup Table3/1
  1-D Lookup Table3/1 -> EngineOFF_PressureController1/1(PUMP SIGNAL 1 - ON)
  BotaoStartStop_b/1 -> Switch/2  "PreStartCondition"
  ChaveDetectada_b/1 -> Switch1/2
  Switch1/1 -> PressaoCombustivel_P/1
  Switch/1 -> Switch1/1

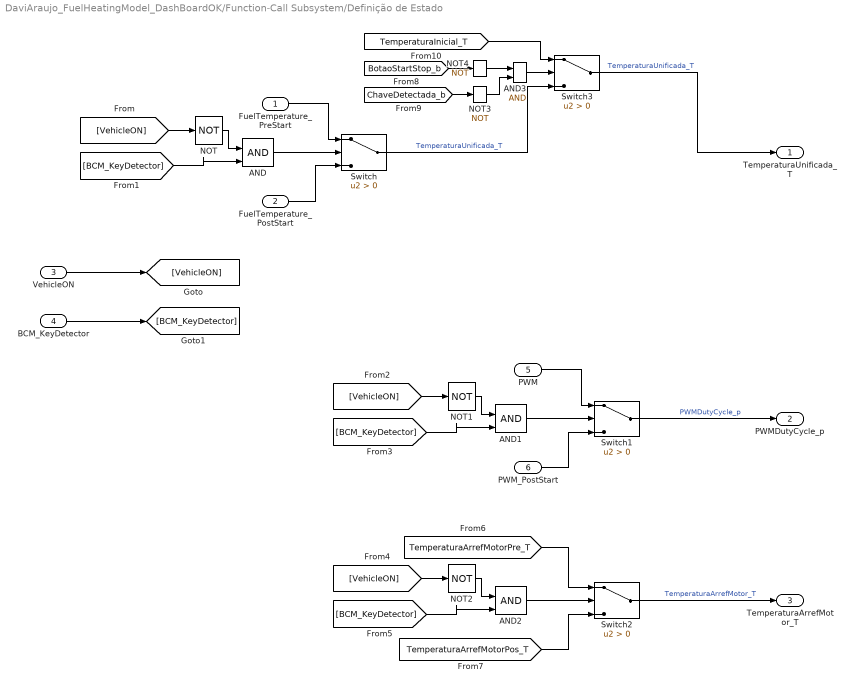
== system DaviAraujo_FuelHeatingModel_DashBoardOK/Function-Call Subsystem/Definição de Estado ==
  FuelTemperature_PreStart : Inport
  FuelTemperature_PostStart : Inport  Port=2
  VehicleON : Inport  Port=3
  BCM_KeyDetector : Inport  Port=4
  PWM : Inport  Port=5
  PWM_PostStart : Inport  Port=6
  AND{,1..3} (4 alike) : Logic  IconShape=distinctive  AllPortsSameDT=off  OutDataTypeStr=boolean
  NOT{,1..4} (5 alike) : Logic  Operator=NOT  IconShape=distinctive  AllPortsSameDT=off  OutDataTypeStr=boolean
  Switch{,1..3} (4 alike) : Switch  Criteria=u2 > Threshold
  TemperaturaUnificada_T : Outport
  PWMDutyCycle_p : Outport  Port=2
  TemperaturaArrefMotor_T : Outport  Port=3
  wires:
  VehicleON/1 -> [VehicleON]
  BCM_KeyDetector/1 -> [BCM_KeyDetector]
  AND/1 -> Switch/2
  [VehicleON] -> NOT/1
  NOT/1 -> AND/1
  [BCM_KeyDetector] -> AND/2
  FuelTemperature_PreStart/1 -> Switch/1
  FuelTemperature_PostStart/1 -> Switch/3
  NOT1/1 -> AND1/1
  [VehicleON] -> NOT1/1
  PWM/1 -> Switch1/1
  PWM_PostStart/1 -> Switch1/3
  [BCM_KeyDetector] -> AND1/2
  AND1/1 -> Switch1/2
  Switch1/1 -> PWMDutyCycle_p/1  "PWMDutyCycle_p"
  NOT2/1 -> AND2/1
  [VehicleON] -> NOT2/1
  [TemperaturaArrefMotorPre_T] -> Switch2/1
  [TemperaturaArrefMotorPos_T] -> Switch2/3
  [BCM_KeyDetector] -> AND2/2
  AND2/1 -> Switch2/2
  Switch2/1 -> TemperaturaArrefMotor_T/1  "TemperaturaArrefMotor_T"
  AND3/1 -> Switch3/2
  [TemperaturaInicial_T] -> Switch3/1
  [ChaveDetectada_b] -> NOT3/1
  Switch/1 -> Switch3/3  "TemperaturaUnificada_T"
  Switch3/1 -> TemperaturaUnificada_T/1  "TemperaturaUnificada_T"
  NOT3/1 -> AND3/2
  [BotaoStartStop_b] -> NOT4/1
  NOT4/1 -> AND3/1

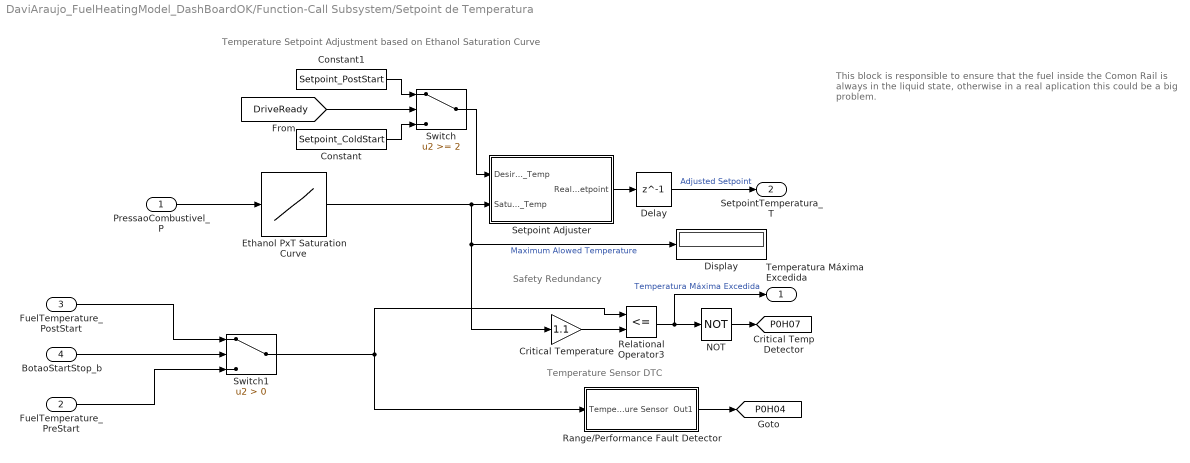
== system DaviAraujo_FuelHeatingModel_DashBoardOK/Function-Call Subsystem/Setpoint de Temperatura ==
  note: Temperature Sensor DTC
  note: Temperature Setpoint Adjustment based on Ethanol Saturation Curve
  note: This block is responsible to ensure that the
      | fuel inside the Comon Rail is always in the liquid state, otherwise in a real aplication this could be a big problem.
  note: Safety Redundancy
  PressaoCombustivel_P : Inport
  FuelTemperature_PreStart : Inport  Port=2
  FuelTemperature_PostStart : Inport  Port=3
  BotaoStartStop_b : Inport  Port=4
  Constant : Constant  Value=Setpoint_ColdStart
  Constant1 : Constant  Value=Setpoint_PostStart
  Critical Temperature : Gain  Gain=1.1
  Delay : Delay  DelayLength=1  InitialCondition=25  SampleTime=0.01
  Display : Display
  Ethanol PxT Saturation Curve : Lookup_n-D  NumberOfTableDimensions=1  BreakpointsForDimension1=Pressure_Ethanol  BreakpointsForDimension2=[1:3]  Table=Temp_Ethanol  InternalRulePriority=Speed  RndMeth=Simplest  InputSameDT=on
  NOT : Logic  Operator=NOT  IconShape=distinctive  AllPortsSameDT=off  OutDataTypeStr=boolean
  Range/Performance Fault Detector : Subsystem
  Relational Operator3 : RelationalOperator  Operator=<=  OutDataTypeStr=boolean  RndMeth=Simplest
  Setpoint Adjuster : Stateflow chart  TreatAsAtomicUnit=on
  Switch : Switch  Threshold=2
  Switch1 : Switch  Criteria=u2 > Threshold
  Temperatura Máxima Excedida : Outport  VectorParamsAs1DForOutWhenUnconnected=off
  SetpointTemperatura_T : Outport  Port=2  VectorParamsAs1DForOutWhenUnconnected=off
  tag scope: P0H04=global, P0H07=global
  wires:
  Setpoint Adjuster/1(Real_Setpoint) -> Delay/1
  NOT/1 -> [P0H07]
  Switch/1 -> Setpoint Adjuster/1(DesiredSetpoint_Temp)
  Constant/1 -> Switch/3
  Range/Performance Fault Detector/1(Out1) -> [P0H04]
  Critical Temperature/1 -> Relational Operator3/2
  [DriveReady] -> Switch/2
  Constant1/1 -> Switch/1
  Relational Operator3/1 -> NOT/1, Temperatura Máxima Excedida/1  "Temperatura Máxima Excedida"
  PressaoCombustivel_P/1 -> Ethanol PxT Saturation Curve/1
  Ethanol PxT Saturation Curve/1 -> Setpoint Adjuster/2(Saturation_Temp), Display/1, Critical Temperature/1  "Maximum Alowed Temperature"
  Delay/1 -> SetpointTemperatura_T/1  "Adjusted Setpoint"
  BotaoStartStop_b/1 -> Switch1/2
  Switch1/1 -> Range/Performance Fault Detector/1(Temperature Sensor), Relational Operator3/1
  FuelTemperature_PostStart/1 -> Switch1/1
  FuelTemperature_PreStart/1 -> Switch1/3

== system DaviAraujo_FuelHeatingModel_DashBoardOK/Function-Call Subsystem/BMS (Chumbo)/Instant Power Consumption1 ==
  Gain : Gain  Gain=(400*4)/(100*3600)
  Out1 : Outport
  wires:
  [PWMDutyCycle_p] -> Gain/1
  Gain/1 -> Out1/1

== system DaviAraujo_FuelHeatingModel_DashBoardOK/Function-Call Subsystem/BMS (Lítio)/Instant Power Consumption1 ==
  Gain : Gain  Gain=(400*4)/(100*3600)
  Out1 : Outport
  wires:
  [PWMDutyCycle_p] -> Gain/1
  Gain/1 -> Out1/1

== system DaviAraujo_FuelHeatingModel_DashBoardOK/Function-Call Subsystem/Condições de Ativação/FuSa 5 ==
  BMS_Lead_SoC : Inport
  BMS_Lead_Temp : Inport  Port=2
  BMS_Lithium_SoC : Inport  Port=3
  BMS_Lithium_Temp : Inport  Port=4
  "Battery Selector " : Stateflow chart  TreatAsAtomicUnit=on
  Constant : Constant  Value=0
  Relational Operator : RelationalOperator  Operator=>  OutDataTypeStr=boolean  RndMeth=Simplest
  Out1 : Outport
  tag scope: BatterySelector=global
  wires:
  BMS_Lead_SoC/1 -> "Battery Selector "/1(BMS_Lead_SoC)
  "Battery Selector "/1(BatterySelector) -> Relational Operator/1, [BatterySelector]
  Constant/1 -> Relational Operator/2
  Relational Operator/1 -> Out1/1
  BMS_Lithium_Temp/1 -> "Battery Selector "/4(BMS_Lithium_Temp)
  BMS_Lead_Temp/1 -> "Battery Selector "/2(BMS_Lead_Temp)
  BMS_Lithium_SoC/1 -> "Battery Selector "/3(BMS_Lithium_SoC)

== system DaviAraujo_FuelHeatingModel_DashBoardOK/Function-Call Subsystem/Condições de Ativação/Malfuncion active ==
  Display : Display
  NOT : Logic  Operator=NOT  IconShape=distinctive  AllPortsSameDT=off  OutDataTypeStr=boolean
  OR : Logic  Operator=OR  Inputs=7  IconShape=distinctive  AllPortsSameDT=off  OutDataTypeStr=boolean
  Malfunction : Outport
  wires:
  OR/1 -> NOT/1
  [P0H07] -> OR/7
  [P0H01] -> OR/1
  [P0H05] -> OR/5
  [P0H02] -> OR/2
  [P0H04] -> OR/4
  [P0H03] -> OR/3
  [P0H06] -> OR/6
  NOT/1 -> Display/1, Malfunction/1

== system DaviAraujo_FuelHeatingModel_DashBoardOK/Function-Call Subsystem/Condições de Ativação/Requirement 1  ==
  note: Ethanol Sensor NORMAL Operation.
  note: Ethanol Sensor DTC.
  ECU_EthanolPercent : Inport
  AND : Logic  IconShape=distinctive  AllPortsSameDT=off  OutDataTypeStr=boolean
  Max E% : Constant  Value=100
  Min E% : Constant  Value=85
  Range/Performance Fault Detector : Subsystem
  Relational Operator : RelationalOperator  OutDataTypeStr=boolean  RndMeth=Simplest
  Relational Operator4 : RelationalOperator  Operator=<=  OutDataTypeStr=boolean  RndMeth=Simplest
  Out1 : Outport  VectorParamsAs1DForOutWhenUnconnected=off
  tag scope: P0H03=global
  wires:
  AND/1 -> Out1/1
  Max E%/1 -> Relational Operator4/2
  Min E%/1 -> Relational Operator/2
  Relational Operator4/1 -> AND/1
  Relational Operator/1 -> AND/2
  ECU_EthanolPercent/1 -> Range/Performance Fault Detector/1(In1), Relational Operator/1, Relational Operator4/1
  Range/Performance Fault Detector/1(Out1) -> [P0H03]

== system DaviAraujo_FuelHeatingModel_DashBoardOK/Function-Call Subsystem/Controlador de Aquecimento Pré Partida/Fuel Mix Specific Fuel Heat ==
  FuelMix_Feedback : Inport
  Specific Heat Etanol : Inport  Port=2
  Specific Heat Gasoline : Inport  Port=3
  Add : Sum  Inputs=+-
  Add1 : Sum
  Constant3 : Constant  Value=100
  Gain : Gain  Gain=-1
  Gain1 : Gain  Gain=1/100
  Product1 : Product
  Product2 : Product
  Specific Heat Mixture : Outport
  wires:
  FuelMix_Feedback/1 -> Add/1, Product1/1
  Gain/1 -> Product2/1
  Add1/1 -> Gain1/1
  Add/1 -> Gain/1
  Constant3/1 -> Add/2
  Product2/1 -> Add1/2
  Specific Heat Etanol/1 -> Product1/2
  Product1/1 -> Add1/1
  Gain1/1 -> Specific Heat Mixture/1
  Specific Heat Gasoline/1 -> Product2/2

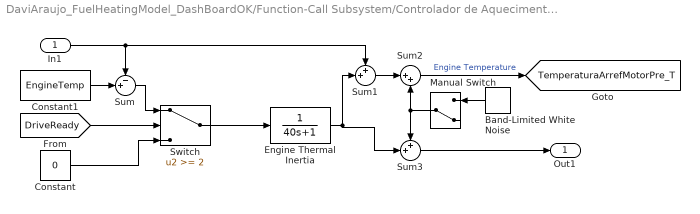
== system DaviAraujo_FuelHeatingModel_DashBoardOK/Function-Call Subsystem/Controlador de Aquecimento Pré Partida/PLANT - Engine Temperature ==
  In1 : Inport
  Band-Limited White Noise : simulink/Sources/Band-Limited White Noise  Cov=[0.001]  Ts=0.05  seed=[23341]
  Constant : Constant  Value=0
  Constant1 : Constant  Value=EngineTemp
  Engine Thermal Inertia : TransferFcn  Denominator=[40 1]
  Manual Switch : ManualSwitch  CurrentSetting=0
  Sum : Sum  Inputs=-+|
  Sum1 : Sum  Inputs=++|
  Sum2 : Sum  Inputs=|++
  Sum3 : Sum  Inputs=++|
  Switch : Switch  Threshold=2
  Out1 : Outport
  tag scope: TemperaturaArrefMotorPre_T=global
  wires:
  Switch/1 -> Engine Thermal Inertia/1
  [DriveReady] -> Switch/2
  Constant/1 -> Switch/3
  Constant1/1 -> Sum/2
  Engine Thermal Inertia/1 -> Sum3/2, Sum1/2
  In1/1 -> Sum1/1, Sum/1
  Sum/1 -> Switch/1
  Sum1/1 -> Sum2/1
  Sum2/1 -> [TemperaturaArrefMotorPre_T]  "Engine Temperature"
  Sum3/1 -> Out1/1
  Manual Switch/1 -> Sum2/2, Sum3/1
  Band-Limited White Noise/1 -> Manual Switch/1

== system DaviAraujo_FuelHeatingModel_DashBoardOK/Function-Call Subsystem/Controlador de Aquecimento Pós Partida/Fuel Mix Specific Fuel Heat ==
  FuelMix_Feedback : Inport
  Specific Heat Etanol : Inport  Port=2
  Specific Heat Gasoline : Inport  Port=3
  Add : Sum  Inputs=+-
  Add1 : Sum
  Constant3 : Constant  Value=100
  Gain : Gain  Gain=-1
  Gain1 : Gain  Gain=1/100
  Product1 : Product
  Product2 : Product
  Specific Heat Mixture : Outport
  wires:
  FuelMix_Feedback/1 -> Add/1, Product1/1
  Gain/1 -> Product2/1
  Add1/1 -> Gain1/1
  Add/1 -> Gain/1
  Constant3/1 -> Add/2
  Product2/1 -> Add1/2
  Specific Heat Etanol/1 -> Product1/2
  Product1/1 -> Add1/1
  Gain1/1 -> Specific Heat Mixture/1
  Specific Heat Gasoline/1 -> Product2/2

== system DaviAraujo_FuelHeatingModel_DashBoardOK/Function-Call Subsystem/Controlador de Aquecimento Pós Partida/PLANT - Engine Temperature ==
  note: This Block emulate the heating behavior of the engine when it starts.
  In1 : Inport
  Band-Limited White Noise : simulink/Sources/Band-Limited White Noise  Cov=[0.001]  Ts=0.05  seed=[23341]
  Constant : Constant  Value=0
  Constant1 : Constant  Value=EngineTemp
  Engine Thermal Inertia : TransferFcn  Denominator=[40 1]
  Manual Switch : ManualSwitch  CurrentSetting=0
  Sum : Sum  Inputs=-+|
  Sum1 : Sum  Inputs=++|
  Sum2 : Sum  Inputs=|++
  Sum3 : Sum  Inputs=++|
  Switch : Switch  Threshold=2
  Engine Temperature Variation : Outport
  tag scope: TemperaturaArrefMotorPos_T=global
  wires:
  Switch/1 -> Engine Thermal Inertia/1
  [DriveReady] -> Switch/2
  Constant/1 -> Switch/3
  Constant1/1 -> Sum/2
  Engine Thermal Inertia/1 -> Sum3/2, Sum1/2
  In1/1 -> Sum1/1, Sum/1
  Sum/1 -> Switch/1
  Sum1/1 -> Sum2/1
  Sum2/1 -> [TemperaturaArrefMotorPos_T]  "Engine Temperature"
  Sum3/1 -> Engine Temperature Variation/1
  Manual Switch/1 -> Sum2/2, Sum3/1
  Band-Limited White Noise/1 -> Manual Switch/1

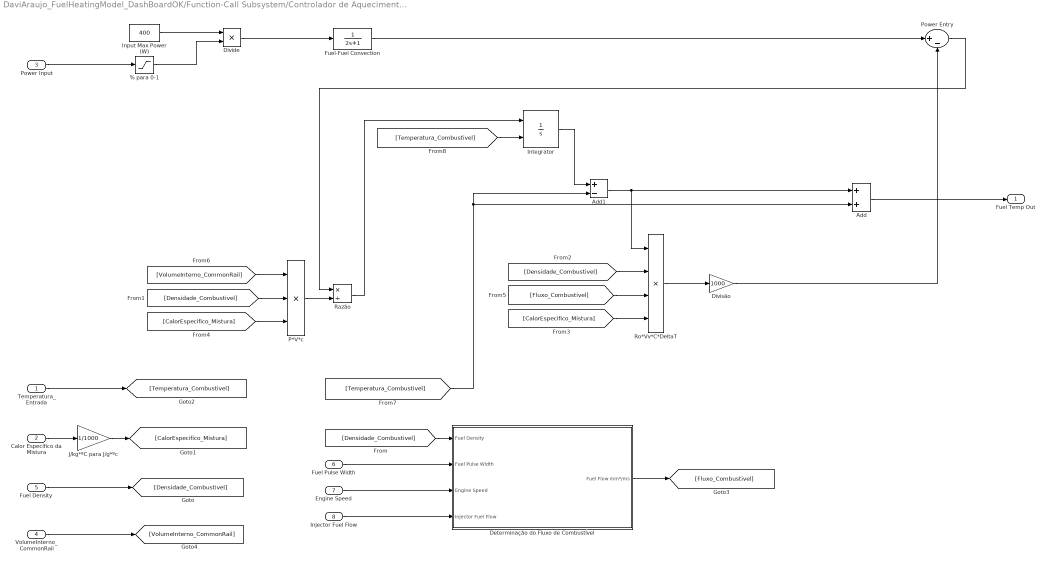
== system DaviAraujo_FuelHeatingModel_DashBoardOK/Function-Call Subsystem/Controlador de Aquecimento Pós Partida/Transient Engine ON - Fuel Heating System ==
  Temperatura_Entrada : Inport
  Calor Específico da Mistura : Inport  Port=2
  Power Input : Inport  Port=3
  VolumeInterno_CommonRail : Inport  Port=4
  Fuel Density : Inport  Port=5
  Fuel Pulse Width : Inport  Port=6
  Engine Speed : Inport  Port=7
  Injector Fuel Flow : Inport  Port=8
  % para 0-1 : Saturate  UpperLimit=1  LowerLimit=0
  Add : Sum
  Add1 : Sum  Inputs=+-
  Determinação do Fluxo de Combustível : Subsystem
  Divide : Product  Inputs=**
  Divisão : Gain  Gain=1000
  Fuel-Fuel Convection : TransferFcn  Denominator=[2 1]
  Input Max Power (W) : Constant  Value=400
  Integrator : Integrator  InitialConditionSource=external
  J/kg*ºC para J/g*ºc : Gain  Gain=1/1000
  P*V*c : Product  Inputs=***
  Power Entry : Sum  Inputs=|+-
  Razão : Product  Inputs=*/
  Ro*Vv*C*DeltaT : Product  Inputs=****
  Fuel Temp Out : Outport
  wires:
  Power Entry/1 -> Razão/1
  Divisão/1 -> Power Entry/2
  P*V*c/1 -> Razão/2
  Razão/1 -> Integrator/1
  Ro*Vv*C*DeltaT/1 -> Divisão/1
  Calor Específico da Mistura/1 -> J/kg*ºC para J/g*ºc/1
  [Temperatura_Combustivel] -> Add1/2, Add/2
  Engine Speed/1 -> Determinação do Fluxo de Combustível/3(Engine Speed)
  Injector Fuel Flow/1 -> Determinação do Fluxo de Combustível/4(Injector Fuel Flow)
  Integrator/1 -> Add1/1
  Add/1 -> Fuel Temp Out/1
  Fuel Pulse Width/1 -> Determinação do Fluxo de Combustível/2(Fuel Pulse Width)
  [Densidade_Combustivel] -> Determinação do Fluxo de Combustível/1(Fuel Density)
  Fuel Density/1 -> [Densidade_Combustivel]
  [Densidade_Combustivel] -> P*V*c/2
  [Densidade_Combustivel] -> Ro*Vv*C*DeltaT/2
  J/kg*ºC para J/g*ºc/1 -> [CalorEspecifico_Mistura]
  [CalorEspecifico_Mistura] -> Ro*Vv*C*DeltaT/4
  [CalorEspecifico_Mistura] -> P*V*c/3
  Determinação do Fluxo de Combustível/1(Fuel Flow mm³/ms) -> [Fluxo_Combustivel]
  [Fluxo_Combustivel] -> Ro*Vv*C*DeltaT/3
  VolumeInterno_CommonRail/1 -> [VolumeInterno_CommonRail]
  [VolumeInterno_CommonRail] -> P*V*c/1
  Temperatura_Entrada/1 -> [Temperatura_Combustivel]
  Add1/1 -> Ro*Vv*C*DeltaT/1, Add/1
  [Temperatura_Combustivel] -> Integrator/2
  Input Max Power (W)/1 -> Divide/1
  Power Input/1 -> % para 0-1/1
  % para 0-1/1 -> Divide/2
  Divide/1 -> Fuel-Fuel Convection/1
  Fuel-Fuel Convection/1 -> Power Entry/1

== system DaviAraujo_FuelHeatingModel_DashBoardOK/Function-Call Subsystem/Controlador de Pressão de Combustível/EngineOFF_PressureController1 ==
  PUMP SIGNAL 1 - ON : Inport
  Atmosphere Pressure : Inport  Port=2
  FUEL PUMP PRESSURE PLANT : TransferFcn  Numerator=[22.5 77.74]  Denominator=[1 11.61 16.21]
  PRESSURE REGULATOR TOPLIMIT : Saturate  UpperLimit=3.28  LowerLimit=0
  Relative To Absolute Pressure : Sum
  Scope : Scope  NumInputPorts=2
  Out1 : Outport
  wires:
  Relative To Absolute Pressure/1 -> Out1/1
  PRESSURE REGULATOR TOPLIMIT/1 -> Relative To Absolute Pressure/1
  PUMP SIGNAL 1 - ON/1 -> Scope/1, FUEL PUMP PRESSURE PLANT/1
  FUEL PUMP PRESSURE PLANT/1 -> Scope/2, PRESSURE REGULATOR TOPLIMIT/1
  Atmosphere Pressure/1 -> Relative To Absolute Pressure/2

== system DaviAraujo_FuelHeatingModel_DashBoardOK/Function-Call Subsystem/Controlador de Pressão de Combustível/EngineON_PressureController1 ==
  PUMP SIGNAL 1 - ON : Inport
  Atmosphere Pressure : Inport  Port=2
  FUEL PUMP PRESSURE PLANT : TransferFcn  Numerator=[22.5 77.74]  Denominator=[1 11.61 16.21]
  PRESSURE REGULATOR TOPLIMIT : Saturate  UpperLimit=3.28  LowerLimit=0
  Relative To Absolute Pressure : Sum
  Scope : Scope  NumInputPorts=2
  Out1 : Outport
  wires:
  Relative To Absolute Pressure/1 -> Out1/1
  PRESSURE REGULATOR TOPLIMIT/1 -> Relative To Absolute Pressure/1
  PUMP SIGNAL 1 - ON/1 -> Scope/1, FUEL PUMP PRESSURE PLANT/1
  FUEL PUMP PRESSURE PLANT/1 -> Scope/2, PRESSURE REGULATOR TOPLIMIT/1
  Atmosphere Pressure/1 -> Relative To Absolute Pressure/2

== system DaviAraujo_FuelHeatingModel_DashBoardOK/Function-Call Subsystem/Setpoint de Temperatura/Range//Performance Fault Detector ==
  Temperature Sensor : Inport
  Below 0% : Constant  Value=-40
  Exceds 100% : Constant  Value=160
  OR : Logic  Operator=OR  IconShape=distinctive  AllPortsSameDT=off  OutDataTypeStr=boolean
  Relational Operator1 : RelationalOperator  Operator=<  OutDataTypeStr=boolean  RndMeth=Simplest
  Relational Operator2 : RelationalOperator  Operator=>  OutDataTypeStr=boolean  RndMeth=Simplest
  Out1 : Outport
  wires:
  Temperature Sensor/1 -> Relational Operator2/1, Relational Operator1/1
  Exceds 100%/1 -> Relational Operator2/2
  Below 0%/1 -> Relational Operator1/2
  Relational Operator2/1 -> OR/1
  Relational Operator1/1 -> OR/2
  OR/1 -> Out1/1

== system DaviAraujo_FuelHeatingModel_DashBoardOK/Function-Call Subsystem/Condições de Ativação/Requirement 1 /Range//Performance Fault Detector ==
  In1 : Inport
  Below 0% : Constant  Value=0
  Exceds 100% : Constant  Value=100
  OR : Logic  Operator=OR  IconShape=distinctive  AllPortsSameDT=off  OutDataTypeStr=boolean
  Relational Operator1 : RelationalOperator  Operator=<  OutDataTypeStr=boolean  RndMeth=Simplest
  Relational Operator2 : RelationalOperator  Operator=>  OutDataTypeStr=boolean  RndMeth=Simplest
  Out1 : Outport
  wires:
  In1/1 -> Relational Operator1/1, Relational Operator2/1
  Exceds 100%/1 -> Relational Operator2/2
  Below 0%/1 -> Relational Operator1/2
  Relational Operator2/1 -> OR/1
  Relational Operator1/1 -> OR/2
  OR/1 -> Out1/1
